simulink model "tesla_motor_testbench_R2019a"  (R2019a)
settings: Solver=VariableStepAuto  StartTime=0.0  StopTime=0.6  RelTol=1e-3
model workspace (MATLAB code in the model file):
  | fsupply = 288;
  | fsupply = 100;
  | V_per_f = 375/288;
  | Vsupply = V_per_f*fsupply;
  | Vsupply = Vsupply + 2; % Voltage boosting
libraries: powerlib x9, powerlib_meascontrol x1, eeSinGeneratorThreePhase x1
settings Model: Creator=kjartan  LastModifiedBy=kjartan

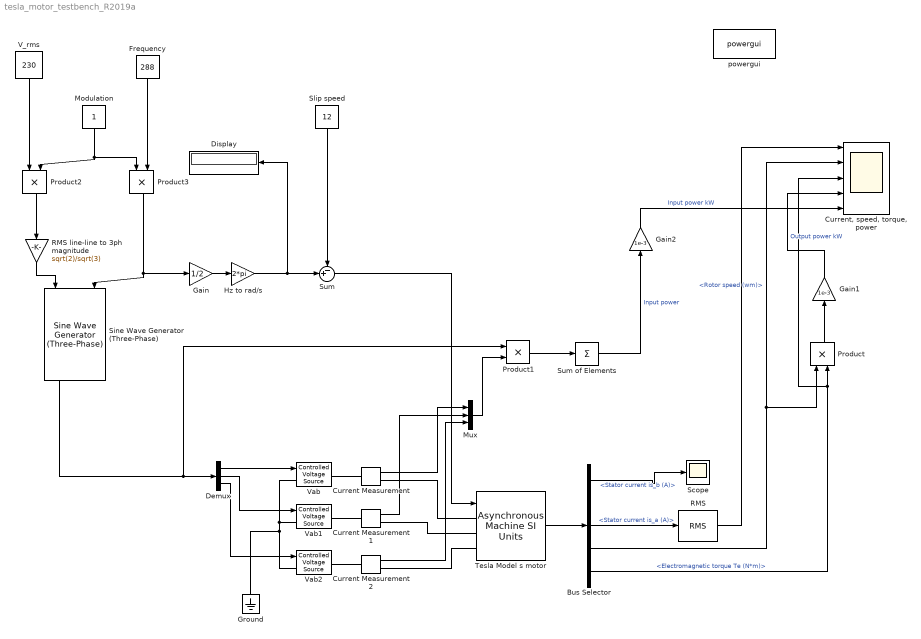
== system tesla_motor_testbench_R2019a ==
  Bus Selector : BusSelector  OutputSignals=Stator measurements.Stator current is_b (A),Stator measurements.Stator current is_c (A),Stator measurements.Stator current is_a (A),Mechanical.Rotor speed (wm),Mechanical.Electromagnetic torque Te (N*m)
  Current Measurement : powerlib/Measurements/Current Measurement  PhasorSimulation=off  OutputType=Complex  PSBequivalent=0
  Current Measurement1 : powerlib/Measurements/Current Measurement  PhasorSimulation=off  OutputType=Complex  PSBequivalent=0
  Current Measurement2 : powerlib/Measurements/Current Measurement  PhasorSimulation=off  OutputType=Complex  PSBequivalent=0
  "Current, speed, torque, power" : Scope  NumInputPorts=5
  Demux : Demux  Outputs=3
  Display : Display
  Frequency : Constant  Value=288
  Gain : Gain  Gain=1/2
  Gain1 : Gain  Gain=1e-3
  Gain2 : Gain  Gain=1e-3
  Ground : powerlib/Elements/Ground  LConnTagsString=a
  Hz to rad/s : Gain  Gain=2*pi
  Modulation : Constant
  Mux : Mux  Inputs=3
  Product{,1..3} (4 alike) : Product
  RMS : powerlib_meascontrol/Measurements/RMS  TrueRMS=on  Freq=60  RMSInit=120  Ts=0
  RMS line-line to 3ph magnitude : Gain  Gain=sqrt(2)/sqrt(3)
  Scope : Scope
  Sine Wave Generator (Three-Phase) : eeSinGeneratorThreePhase/Sine Wave Generator (Three-Phase)  Ts=1/(40*288)
      settings: SourceProductBaseCode=PS
  Slip speed : Constant  Value=12
  Sum : Sum  Inputs=-+|
  Sum of Elements : Sum  Inputs=+
  Tesla Model s motor : powerlib/Machines/Asynchronous Machine SI Units  RotorType=Squirrel-cage  PresetModel=No  MechanicalLoad=Speed w  ShowDetailedParameters=on  ReferenceFrame=Rotor  Units=SI  MeasurementBus=off  NominalParameters=[375, 230, 288]  Stator=[3e-3, 1.38e-6]  Rotor=[2e-3, 1.1052e-5]  Cage1=[0.4155 0.002066]  Cage2=[0.4168 0.0003495]  Lm=0.33157e-3  Mechanical=[0.05 0.005879 2]  PolePairs=2  InitialConditions=[0 0 0 0 0 0 0 0]  SimulateSaturation=off  Saturation=[14.03593122, 27.81365428, 53.79336849, 72.68890987, 97.98006896, 148.6815601, 215.7428561, 302.9841135, 428.7778367 ; 230, 322, 414, 460, 506, 552, 598, 644, 690]  LoadFlowParameters=1492000  TsPowergui=0  TsBlock=-1  IterativeModel=Trapezoidal non iterative  IterativeDiscreteModel=Trapezoidal non iterative  Pmec=1.492e+006
  V_rms : Constant  Value=230
  Vab : powerlib/Electrical Sources/Controlled Voltage Source  Description=source block  Initialize=on  Source_Type=AC  Amplitude=0  Phase=0  Frequency=0  Measurements=None
      settings: AttributesFormatString=\n
  Vab1 : powerlib/Electrical Sources/Controlled Voltage Source  Description=source block  Initialize=on  Source_Type=AC  Amplitude=0  Phase=0  Frequency=0  Measurements=None
      settings: AttributesFormatString=\n
  Vab2 : powerlib/Electrical Sources/Controlled Voltage Source  Description=source block  Initialize=on  Source_Type=AC  Amplitude=0  Phase=0  Frequency=0  Measurements=None
      settings: AttributesFormatString=\n
  powergui : powerlib/powergui  Priority=1  SimulationMode=Continuous  SampleTime=50e-6  frequency=60  Iterations=50  frequencyindice=0  Pbase=100e6  ErrMax=1e-4  UnitsV=kV  UnitsW=MW  buscounter=0  FunctionMessages=off  echomessages=off  EnableUseOfTLC=off  CurrentSourceSwitches=off  DisableSnubberDevices=off  DisableRonSwitches=off  DisableVfSwitches=off  DisplayEquations=off  AutomaticDiscreteSolvers=off  SolverType=Tustin/Backward Euler (TBE)  Interpol=off  ExternalGateDelay=off  methode=off  Ts=100  x0status=blocks  SPID=on  SwTol=0  HookPort=off  NonlinearTolerance=1e-4  nMaxIteration=100  ContinueOnMaxIteration=off  RestoreLinks=warning  ResistiveCurrentMeasurement=off  Frange=[0:2:500]  Ylog=off  Xlog=on  ShowGrid=off  save=off  variable=ZData  structure=0  ZoomFFT=off  StartTime=0.0  cycles=1  DisplayStyle=1  fundamental=60  FreqAxis=off  MaxFrequency=1000  frequencyindicesteady=1  RmsSteady=1  display=off
  wires:
  Slip speed/1 -> Sum/1
  Hz to rad/s/1 -> Display/1, Sum/2
  Gain/1 -> Hz to rad/s/1
  Product/1 -> Gain1/1
  Gain1/1 -> "Current, speed, torque, power"/4  "Output power kW"
  Product1/1 -> Sum of Elements/1
  Sum of Elements/1 -> Gain2/1  "Input power"
  Gain2/1 -> "Current, speed, torque, power"/5  "Input power kW"
  RMS line-line to 3ph magnitude/1 -> Sine Wave Generator (Three-Phase)/1
  Bus Selector/1 -> Scope/1  "<Stator current is_b (A)>"
  Demux/3 -> Vab2/1
  Demux/1 -> Vab/1
  Demux/2 -> Vab1/1
  Tesla Model s motor/1 -> Bus Selector/1
  Sine Wave Generator (Three-Phase)/1 -> Product1/1, Demux/1
  Sum/1 -> Tesla Model s motor/1
  Bus Selector/3 -> RMS/1  "<Stator current is_a (A)>"
  Bus Selector/4 -> Product/1, "Current, speed, torque, power"/2  "<Rotor speed (wm)>"
  Bus Selector/5 -> "Current, speed, torque, power"/3, Product/2  "<Electromagnetic torque Te (N*m)>"
  RMS/1 -> "Current, speed, torque, power"/1
  Current Measurement/1 -> Mux/1
  Current Measurement1/1 -> Mux/2
  Current Measurement2/1 -> Mux/3
  Mux/1 -> Product1/2
  V_rms/1 -> Product2/1
  Product2/1 -> RMS line-line to 3ph magnitude/1
  Frequency/1 -> Product3/2
  Product3/1 -> Sine Wave Generator (Three-Phase)/3, Gain/1
  Modulation/1 -> Product3/1, Product2/2
  connections:
  Vab/LConn1 -- Ground/LConn1 -- Vab2/LConn1 -- Vab1/LConn1
  Vab1/RConn1 -- Current Measurement1/LConn1
  Vab2/RConn1 -- Current Measurement2/LConn1
  Vab/RConn1 -- Current Measurement/LConn1
  Tesla Model s motor/LConn1 -- Current Measurement/RConn1
  Current Measurement1/RConn1 -- Tesla Model s motor/LConn2
  Current Measurement2/RConn1 -- Tesla Model s motor/LConn3
